simulink model "DT_UDE"  (R2019b)
settings: Solver=ode4  StartTime=0.0  StopTime=tstop  FixedStep=tstep  RelTol=1e-3
values from neighbouring files (symbols this model uses):
  tstep = 0.01    [data.m]
  xic = [-2 1]    [data.m]
settings Model: Creator=Ram Padmanabhan  LastModifiedBy=Ram Padmanabhan
settings DataIOCC: SaveOutput=off  SignalLogging=off  DSMLogging=off  SaveTime=off  ReturnWorkspaceOutputs=off

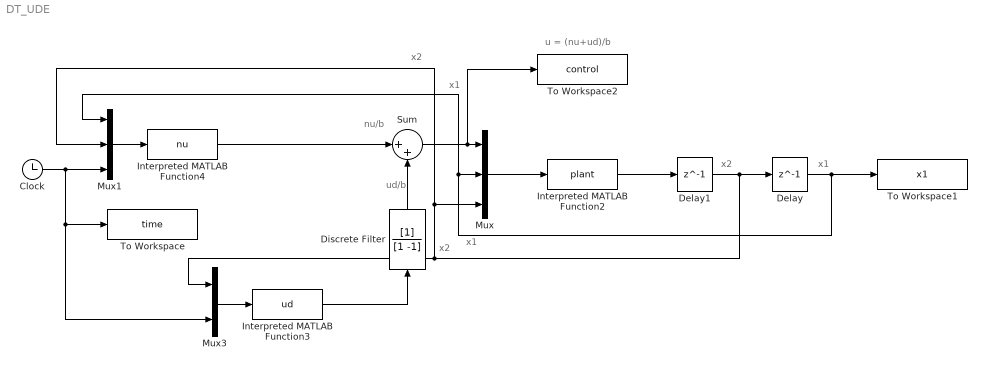
== system DT_UDE ==
  note: u = (nu+ud)/b
  note: ud/b
  note: nu/b
  note: x2
  note: x1
  note: x2
  note: x1
  note: x1
  note: x2
  Clock : Clock
  Delay : Delay  DelayLength=1  InitialCondition=xic(1)  SampleTime=tstep
  Delay1 : Delay  DelayLength=1  InitialCondition=xic(2)  SampleTime=tstep
  Discrete Filter : DiscreteFilter  Denominator=[1 -1]  SampleTime=tstep
  Interpreted MATLAB Function2 : MATLABFcn  MATLABFcn=plant  OutputDimensions=1
  Interpreted MATLAB Function3 : MATLABFcn  MATLABFcn=ud  OutputDimensions=1
  Interpreted MATLAB Function4 : MATLABFcn  MATLABFcn=nu  OutputDimensions=1
  Mux : Mux  Inputs=3
  Mux1 : Mux  Inputs=3
  Mux3 : Mux  Inputs=2
  Sum : Sum  Inputs=|++
  To Workspace : ToWorkspace  VariableName=time  SampleTime=-1
  To Workspace1 : ToWorkspace  VariableName=x1  SampleTime=-1
  To Workspace2 : ToWorkspace  VariableName=control  SampleTime=-1
  wires:
  Delay1/1 -> Mux1/2, Mux/3, Mux3/1, Delay/1
  Interpreted MATLAB Function2/1 -> Delay1/1
  Mux/1 -> Interpreted MATLAB Function2/1
  Delay/1 -> To Workspace1/1, Mux1/1, Mux/2
  Sum/1 -> To Workspace2/1, Mux/1
  Mux1/1 -> Interpreted MATLAB Function4/1
  Clock/1 -> Mux1/3, To Workspace/1, Mux3/2
  Mux3/1 -> Interpreted MATLAB Function3/1
  Interpreted MATLAB Function3/1 -> Discrete Filter/1
  Interpreted MATLAB Function4/1 -> Sum/1
  Discrete Filter/1 -> Sum/2
